simulink model "RK_T22"  (R2018a)
settings: Solver=ode45  StartTime=0.0  StopTime=25  RelTol=1e-3  EnableMultiTasking=on
model workspace (MATLAB code in the model file):
  | Ks = 1.5;
  | T = 1.73; % s
  | D = 1.15;
  | % - - - - - - - - - - -
  | Kkrit = 22.6;
  | Tkrit = 1.93; % s
  | T0 = 0.25; % s
  | % - - - - - - - - - - -
  | Kp = 0.6*Kkrit*(1-T0/Tkrit);
  | T0Tn = 1.2*Kkrit*T0/(Kp*Tkrit); % s
  | TvT0 = 3*Kkrit*Tkrit/(40*Kp*T0); % s
  | % - - - - - - - - - - -
  | p1 = -1;
  | q0 = Kp*(1+T0Tn+TvT0);
  | q1 = -Kp*(1+2*TvT0);
  | q2 = Kp*TvT0;
Description:
  | Regelkreis mit kontinuierlichem PID-Regler
settings Model: ExtModeAutoUpdateStatusClock=off  Creator=manfred  LastModifiedBy=manfred
settings DataIOCC: LimitDataPoints=on  SaveFormat=Array  SignalLoggingSaveFormat=ModelDataLogs  SignalLoggingName=sigsOut
settings OptimizationCC: ExpressionDepthLimit=2147483647  LifeSpan=inf
settings DebuggingCC: SaveWithParameterizedLinksMsg=none  UnderspecifiedInitializationDetection=Classic  MergeDetectMultiDrivingBlocksExec=none  SignalResolutionControl=TryResolveAllWithWarning  MultiTaskDSMMsg=warning  MultiTaskCondExecSysMsg=none  FcnCallInpInsideContextMsg=warning  StateNameClashWarn=warning  SFUnexpectedBacktrackingDiag=warning  SFNoUnconditionalDefaultTransitionDiag=warning  SFExecutionAtInitializationDiag=none
settings HardwareCC: ProdBitPerPointer=32  ProdBitPerSizeT=32  ProdBitPerPtrDiffT=32  ProdLargestAtomicFloat=None  ProdIntDivRoundTo=Undefined  ProdEndianess=Unspecified  ProdWordSize=32  ProdHWDeviceType=32-bit Generic  TargetUnknown=on
settings ModelReferenceCC: PropagateSignalLabelsOutOfModel=off
settings CodeAppCC: StateflowObjectComments=on
settings GRTTargetCC: TargetLangStandard=C89/C90 (ANSI)  CombineOutputUpdateFcns=off  GRTInterface=on
settings ConfigComp: CovMetricSettings=dw  CovHtmlReporting=on  CovSaveCumulativeToWorkspaceVar=on  CovSaveSingleToWorkspaceVar=on  CovExternalEMLEnable=off

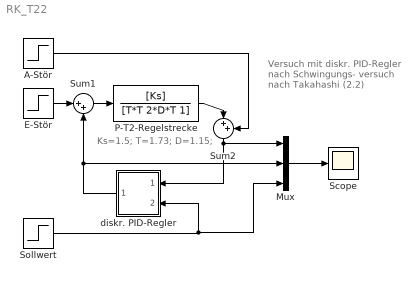
== system RK_T22 ==
  note: Ks=1.5; T=1.73; D=1.15;
  note: Versuch mit diskr.
      | PID-Regler nach
      | Schwingungs-
      | versuch nach
      | Takahashi (2.2)
  A-Stör : Step  Time=15  SampleTime=0
  E-Stör : Step  Time=8  SampleTime=0
  Mux : Mux  Inputs=3
  P-T2-Regelstrecke : TransferFcn  Numerator=[Ks]  Denominator=[T*T 2*D*T 1]  ContinuousStateAttributes='Regelstrecke'
  Scope : Scope
  Sollwert : Step  SampleTime=0
  Sum1 : Sum  Inputs=|++
  Sum2 : Sum  Inputs=|++
  diskr. PID-Regler : Subsystem
  wires:
  Mux/1 -> Scope/1
  Sum1/1 -> P-T2-Regelstrecke/1
  Sum2/1 -> diskr. PID-Regler/1(In1), Mux/1
  P-T2-Regelstrecke/1 -> Sum2/1
  E-Stör/1 -> Sum1/1
  A-Stör/1 -> Sum2/2
  diskr. PID-Regler/1(Out1) -> Sum1/2, Mux/2
  Sollwert/1 -> Mux/3, diskr. PID-Regler/2(In2)

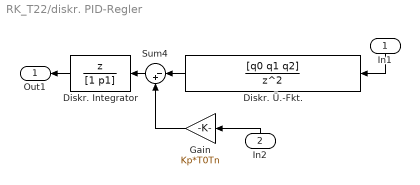
== system RK_T22/diskr. PID-Regler ==
  In1 : Inport
  In2 : Inport  Port=2
  Diskr. Integrator : DiscreteTransferFcn  Numerator=[1 0]  Denominator=[1 p1]  SampleTime=T0
  Diskr. Ü.-Fkt. : DiscreteTransferFcn  Numerator=[q0 q1 q2]  Denominator=[1 0 0]  SampleTime=T0
  Gain : Gain  Gain=Kp*T0Tn
  Sum4 : Sum  Inputs=|-+
  Out1 : Outport
  wires:
  Sum4/1 -> Diskr. Integrator/1
  Diskr. Ü.-Fkt./1 -> Sum4/1
  In1/1 -> Diskr. Ü.-Fkt./1
  Diskr. Integrator/1 -> Out1/1
  Gain/1 -> Sum4/2
  In2/1 -> Gain/1
